simulink model "PubIfDecisionTOS_MDL"  (R2020b)
settings: configuration reference "DspaceConfig" (kept outside this file)
PostLoadFcn:
  | if any(exist('dsrtsu_mdlpostloadfcn', 'file') ~= 0), dsrtsu_mdlpostloadfcn('Execute', bdroot); end
InitFcn:
  | , if any(exist('dsmpb_private', 'file') ~= 0), dsmpb_private('dsmpb_mdlclblib', 'Init', bdroot); end,
undefined symbols (not defined in the file or in its folder): C_TOS_ACCEgoRAxletoFbumplength_m, C_TOS_ACCTargetFront_Flag, C_TOS_AEBJAPedObjDxThre_Val, C_TOS_AEBJAPedObjDyThre_Val, C_TOS_AEBJATargetSize_Val, C_TOS_AEBJAVehObjDxThre_Val, C_TOS_AEBJAVehObjDyThre_Val, C_TOS_AEBJuncPedTargetSize_Val, C_TOS_AEBLatObjDxThre_Val, C_TOS_AEBLatPedDyThre_Val, C_TOS_AEBLatTargetSize_Val, C_TOS_AEBLongTargetInEgoFront_Flag, C_TOS_axAbsGround_Parameter, C_TOS_CameraConfirmedFlag, C_TOS_CNsubjWidth, C_TOS_CurrentLaneCoreMinWidth_Val, C_TOS_CutInProb_Val_Zero, C_TOS_CutOutProb_Val_Zero, C_TOS_D2R_Val, C_TOS_DefaultValueObjectToCenterLine_dy, C_TOS_EgoCarWidth_Val, C_TOS_EgoDxRefPoint_m, C_TOS_EgoRAxletoFbumplength_m, C_TOS_HalfWidthVehicle_Con, C_TOS_HWA_CurrentLaneFlag, C_TOS_HWA_LeftLaneFlag, C_TOS_HWA_MovingDir_Vaild, C_TOS_HWA_MovState_Vaild, C_TOS_HWA_RightLaneFlag, C_TOS_LaneLineCourseErrorFront, C_TOS_LaneLineCourseErrorRear, C_TOS_MotorbikeDefaultWidth_m, C_TOS_NumberOfEffectiveTargets, C_TOS_Obj_Age_Val, C_TOS_Objdx_Constraint_Val, C_TOS_ObjectDefaultWidth_m, C_TOS_ObjInCurrentLane_Val, C_TOS_ObjInCurrentLaneValid, C_TOS_ObjInLeftLaneValid, C_TOS_ObjInRightLaneValid, C_TOS_ObjNotInCurrentLane_Val, C_TOS_ObjNotREElementType, C_TOS_ObjPredictDis_dy_ConstantVal_Zeros, C_TOS_ObjToCenterLine_ConstantVal_Zeros, C_TOS_OFMObjIDInvilad_Val, C_TOS_PIL_LatDisCons_Val_zero, C_TOS_PIL_ObjectCutInFlag_b, C_TOS_PIL_ObjectCutOutFlag_b, C_TOS_PIL_ObjLaneProb_al_Val, C_TOS_PP_ObjFusType_FC_Confirm_b, C_TOS_PP_ObjFusType_FC_FR_Confirm_b, C_TOS_PP_ObjFusType_FR_Confirm_b, C_TOS_RE_80BoolDefault_Val, C_TOS_RE_80Single181Default_Val, C_TOS_RE_80Single255Default_Val, C_TOS_RE_80Uint8Default_Val, C_TOS_RE_D2R, C_TOS_RE_D_180_Val, C_TOS_RE_InvalidObjectID_Val, C_TOS_RE_InvalidTargetChainDir_Val ... (+142)
libraries: simulink x1650, TOS_LIB x361, canfdmsglib x14
(part 8 of 69)

== system PubIfDecisionTOS_MDL/TOS_20201112/TOS_2012080320/TOS/AEB/TOS_AEBLatCro_20201208 ==
  TOSAAt_OFM_TIL_VIE : Inport
  AEBLatTrgInfor : Subsystem
  AEBLat_Object_Condition : Subsystem
  AEBLat_Object_Condition2 : Subsystem  Commented=on
  AEBLat_TargetIndex : Subsystem
  Bus Creator : BusCreator  Inputs=4
  Bus Selector1 : BusSelector  OutputSignals=OFM_SignalVerification.Object_ID,TOS_AddAttributes.PP_ObjFusType_FC_FR_Confirm,TOS_AddAttributes.PP_ObjFusType_FR_Confirm,OFM_SignalVerification.Object_Type,OFM_SignalVerification.Object_DX,OFM_SignalVerification.Object_DY,TOS_AddAttributes.PP_ObjMovingDirSignalProcessing,OFM_SignalVerification.Object_HeadingAngle,OFM_SignalVerification.Object_VX,OFM_SignalVerification.Object_VY,VIE_SignalVerification.vxvRefMs,VIE_SignalVerification.psiDtOpt
  Bus Selector2 : BusSelector  OutputSignals=OFM_SignalVerification,TOS_AddAttributes
  Bus Selector4 : BusSelector  Commented=on  OutputSignals=OFM_SignalVerification.Object_ID,TOS_AddAttributes.PP_ObjFusType_FC_FR_Confirm,TOS_AddAttributes.PP_ObjFusType_FR_Confirm,OFM_SignalVerification.Object_Type,OFM_SignalVerification.Object_DX,OFM_SignalVerification.Object_DY,TOS_AddAttributes.PP_ObjMovingDirSignalProcessing,OFM_SignalVerification.Object_HeadingAngle,OFM_SignalVerification.Object_VX,OFM_SignalVerification.Object_VY,VIE_SignalVerification.vxvRefMs,VIE_SignalVerification.psiDtOpt
  Display{5..9} (5 alike) : Display  Commented=on
  From2 : From  Commented=on  GotoTag=TOS_AEB_LATOBJ
  Selector{10..19} (10 alike) : Selector  Commented=on  InputPortWidth=80  IndexOptions=Index vector (dialog)  Indices=64  OutputSizes=1
  Subsystem : Subsystem
  Subsystem1 : Subsystem
  Subsystem2 : Subsystem  Commented=on
  Terminator : Terminator
  Unit Delay{,1,3..4} (4 alike) : UnitDelay  SampleTime=-1  HasFrameUpgradeWarning=on
  Unit Delay2 : UnitDelay  Commented=on  SampleTime=-1  HasFrameUpgradeWarning=on
  TOS_AEB_LATOBJ : Outport
  wires:
  Bus Selector1/3 -> AEBLat_Object_Condition/3(PP_ObjFusType_FR_Confirm)  "<PP_ObjFusType_FR_Confirm>"
  Bus Selector1/2 -> AEBLat_Object_Condition/2(PP_ObjFusType_FC_FR_Confirm)  "<PP_ObjFusType_FC_FR_Confirm>"
  Bus Selector1/11 -> AEBLat_Object_Condition/11(VIE_EgoVelocity)  "<vxvRefMs>"
  Bus Selector1/10 -> AEBLat_Object_Condition/10(Object_VY)  "<Object_VY>"
  Bus Selector1/9 -> AEBLat_Object_Condition/9(Object_VX)  "<Object_VX>"
  Bus Selector1/8 -> AEBLat_Object_Condition/8(Object_HeadingAngle)  "<Object_HeadingAngle>"
  Bus Selector1/7 -> AEBLat_Object_Condition/7(PP_ObjMovingDirSignalProcessing)  "<PP_ObjMovingDirSignalProcessing>"
  Bus Selector1/1 -> AEBLat_Object_Condition/1(Object_ID)  "<Object_ID>"
  Bus Selector1/4 -> AEBLat_Object_Condition/4(ObjectType)  "<Object_Type>"
  Bus Selector2/1 -> AEBLatTrgInfor/1(OFM_SignalVerification)  "<OFM_SignalVerification>"
  Bus Selector2/2 -> AEBLatTrgInfor/2(TOS_AddAttributes)  "<TOS_AddAttributes>"
  Bus Selector1/5 -> AEBLat_Object_Condition/5(Object_Dx)  "<Object_DX>"
  Bus Selector1/6 -> AEBLat_Object_Condition/6(Object_Dy)  "<Object_DY>"
  AEBLat_TargetIndex/1(AEBLat_Target_Index) -> AEBLatTrgInfor/3(TOS_AEBLatTrg_Index)  "TOS_AEBLat_Index"
  AEBLat_Object_Condition/1(TOS_AEBLat_ConditionTargets_Dx) -> AEBLat_TargetIndex/1(TOS_AEBLat_Targets_Dx)  "TOS_AEBLat_ConditionTargets_Dx"
  AEBLat_Object_Condition/2(AEBLat_TargetFusionType_observal) -> Bus Creator/1  "TOS_AEBLat_TargetFusionType_observal"
  AEBLat_Object_Condition/3(AEBLat_TargetObjectType_observal) -> Bus Creator/2  "TOS_AEBLat_TargetObjectType_observal"
  AEBLat_Object_Condition/4(AEBLat_TargetDXDY_observal) -> Bus Creator/3  "TOS_AEBLat_TargetDXDY_observal"
  AEBLat_Object_Condition/5(AEBLat_TargetMovDir_observal) -> Bus Creator/4  "TOS_AEBLat_TargetMovDir_observal"
  AEBLatTrgInfor/1(TOS_AEB_LATOBJ) -> [TOS_AEB_LATOBJ], TOS_AEB_LATOBJ/1
  Bus Selector1/12 -> AEBLat_Object_Condition/12(psiDtOpt)  "<psiDtOpt>"
  [TOS_AEB_LATOBJ] -> Subsystem/1(TOS_AEB_LATOBJ)
  Subsystem/1(ObjectID) -> Unit Delay/1
  Unit Delay/1 -> AEBLat_Object_Condition/13(AEBLat_Target_ObjectID_K1)
  Selector18/1 -> AEBLat_Object_Condition2/9(Object_VX)
  Selector19/1 -> AEBLat_Object_Condition2/10(Object_VY)
  Selector16/1 -> AEBLat_Object_Condition2/7(PP_ObjMovingDirSignalProcessing)
  Selector17/1 -> AEBLat_Object_Condition2/8(Object_HeadingAngle)
  Selector15/1 -> AEBLat_Object_Condition2/6(Object_Dy)
  Selector14/1 -> AEBLat_Object_Condition2/5(Object_Dx)
  Selector13/1 -> AEBLat_Object_Condition2/4(ObjectType)
  Selector12/1 -> AEBLat_Object_Condition2/3(PP_ObjFusType_FR_Confirm)
  Selector11/1 -> AEBLat_Object_Condition2/2(PP_ObjFusType_FC_FR_Confirm)
  Selector10/1 -> AEBLat_Object_Condition2/1(Object_ID)
  Bus Selector4/3 -> Selector12/1  "<PP_ObjFusType_FR_Confirm>"
  Bus Selector4/2 -> Selector11/1  "<PP_ObjFusType_FC_FR_Confirm>"
  Bus Selector4/11 -> AEBLat_Object_Condition2/11(VIE_EgoVelocity)  "<vxvRefMs>"
  Bus Selector4/10 -> Selector19/1  "<Object_VY>"
  Bus Selector4/9 -> Selector18/1  "<Object_VX>"
  Bus Selector4/8 -> Selector17/1  "<Object_HeadingAngle>"
  Bus Selector4/7 -> Selector16/1  "<PP_ObjMovingDirSignalProcessing>"
  Bus Selector4/1 -> Selector10/1  "<Object_ID>"
  Bus Selector4/4 -> Selector13/1  "<Object_Type>"
  Bus Selector4/5 -> Selector14/1  "<Object_DX>"
  Bus Selector4/6 -> Selector15/1  "<Object_DY>"
  TOSAAt_OFM_TIL_VIE/1 -> Bus Selector2/1, Bus Selector4/1, Bus Selector1/1
  Bus Selector4/12 -> AEBLat_Object_Condition2/12(psiDtOpt)  "<psiDtOpt>"
  From2/1 -> Subsystem2/1(TOS_AEB_LATOBJ)
  Subsystem2/1(ObjectID) -> Unit Delay2/1
  Unit Delay2/1 -> AEBLat_Object_Condition2/13(AEBLat_Target_ObjectID_K1)
  AEBLat_Object_Condition2/5(AEBLat_TargetMovDir_observal) -> Display9/1
  AEBLat_Object_Condition2/4(AEBLat_TargetDXDY_observal) -> Display8/1
  AEBLat_Object_Condition2/3(AEBLat_TargetObjectType_observal) -> Display7/1
  AEBLat_Object_Condition2/2(AEBLat_TargetFusionType_observal) -> Display6/1
  AEBLat_Object_Condition2/1(TOS_AEBLat_ConditionTargets_Dx) -> Display5/1
  Subsystem/2(ObjectType) -> Unit Delay3/1
  Unit Delay3/1 -> AEBLat_Object_Condition/14(AEBLat_Target_ObjectType_K1)
  Unit Delay4/1 -> AEBLatTrgInfor/5(AEBLat_Target_ObjectType_K1)
  Subsystem1/2(ObjectType) -> Unit Delay4/1
  Unit Delay1/1 -> AEBLatTrgInfor/4(AEBLat_Target_ObjectID_K1)
  Subsystem1/1(ObjectID) -> Unit Delay1/1
  [TOS_AEB_LATOBJ] -> Subsystem1/1(TOS_AEB_LATOBJ)
  Bus Creator/1 -> Terminator/1  "TOS_AEBLat_ObserVal"

== system PubIfDecisionTOS_MDL/TOS_20201112/TOS_2012080320/TOS/AEB/TOS_AEBLong ==
  note: 目标分裂，去除Dx2米之内的分裂目标
  TOSAAt_OFM_TIL_VIE : Inport
  AEBLongTargetInfor : Subsystem
  AEBLong_Confirm : Subsystem
  AEBLong_Target_PreJudge : Subsystem
  Bus Selector : BusSelector  OutputSignals=ObjectID,dx
  Bus Selector2 : BusSelector  OutputSignals=OFM_SignalVerification,TOS_AddAttributes
  Bus Selector3 : BusSelector  OutputSignals=OFM_SignalVerification.Object_DX,OFM_SignalVerification.Object_ID,TLJ_TargetInLaneValidityJudg.TOS_TLJ_SameLaneConfirm_Flag
  Bus Selector4 : BusSelector  OutputSignals=VIE_SignalVerification.vxvRefMs,OFM_SignalVerification,TOS_AddAttributes,TLJ_TargetInLaneValidityJudg,PP_CenterLineCalculat,TOS_ProbInLaneCalculat,TOS_VCAN_SignalVerification,TOS_ProbInLaneCalculat.PIL_OverlapRatio
  Bus Selector5 : BusSelector  OutputSignals=TOS_AddAttributes.PP_ObjFusType_FC_FR_Confirm,TOS_AddAttributes.PP_ObjFusType_FR_Confirm,TOS_AddAttributes.PP_ObjFusType_FC_Confirm,OFM_SignalVerification.Object_ID,OFM_SignalVerification.Object_MovingState,OFM_SignalVerification.Object_DX,OFM_SignalVerification.Object_ObstacleProb,OFM_SignalVerification.Object_DY,PP_REElementType
  Bus Selector6 : BusSelector  OutputSignals=ObjectID,ObjectMovingState
  Constant2 : Constant  Value=C_TOS_NumberOfEffectiveTargets  OutDataTypeStr=uint8
      settings: AttributesFormatString=C_TOS_NumberOfEffectiveTargets = 80
  Delay : Delay  InitialCondition=0
  Delay1 : Delay  DelayLength=1  InitialCondition=0
  Delay2 : Delay  InitialCondition=0
  Delay3 : Delay  DelayLength=1  InitialCondition=0
  MATLAB Function1 : MATLAB Function  TreatAsAtomicUnit=on
  MATLAB Function2 : MATLAB Function  Commented=on  TreatAsAtomicUnit=on
  Terminator : Terminator
  Terminator1 : Terminator
  Terminator2 : Terminator
  Unit Delay : UnitDelay  SampleTime=-1  HasFrameUpgradeWarning=on
  Unit Delay1 : UnitDelay  InitialCondition=255  SampleTime=-1  HasFrameUpgradeWarning=on
  TOS_AEBLONOBJ : Outport
  wires:
  Bus Selector4/4 -> AEBLong_Confirm/4(TLJ_TargetInLaneValidityJudg)  "<TLJ_TargetInLaneValidityJudg>"
  Bus Selector4/3 -> AEBLong_Confirm/3(TOS_AddAttributes)  "<TOS_AddAttributes>"
  Bus Selector4/2 -> AEBLong_Confirm/2(OFM_SignalVerification)  "<OFM_SignalVerification>"
  Bus Selector4/1 -> AEBLong_Confirm/1(VIE_EgoVelocity)  "<vxvRefMs>"
  Bus Selector2/2 -> AEBLongTargetInfor/2(TOS_AddAttributes)  "<TOS_AddAttributes>"
  AEBLongTargetInfor/1(TOS_AEBLONOBJ) -> [TOS_AEBLONOBJ], TOS_AEBLONOBJ/1
  Bus Selector2/1 -> AEBLongTargetInfor/1(OFM_SignalVerification)  "<OFM_SignalVerification>"
  AEBLong_Confirm/1(TOS_AEBLong_TargetIndex) -> AEBLongTargetInfor/3(TOS_AEBLongTargetIndex)
  Bus Selector4/5 -> AEBLong_Confirm/5(PP_CenterLineCalculat)  "<PP_CenterLineCalculat>"
  Bus Selector4/6 -> AEBLong_Confirm/6(PIL_ProbInLaneCalculat)  "<TOS_ProbInLaneCalculat>"
  Bus Selector4/7 -> AEBLong_Confirm/7(<TOS_VCAN_SignalVerification>)  "<TOS_VCAN_SignalVerification>"
  Bus Selector3/1 -> MATLAB Function1/1(Object_Dx)  "<Object_DX>"
  Bus Selector3/2 -> MATLAB Function1/2(Object_ID)  "<Object_ID>"
  MATLAB Function1/1(Dx1stNearestObjIndex) -> AEBLong_Confirm/9(AEBLong_Index)  "TOS_AEBLong_Index"
  MATLAB Function1/2(Dx1stNearestObjID) -> Terminator/1
  MATLAB Function1/3(Dx2edNearestObjIndex) -> Terminator1/1
  MATLAB Function1/4(Dx2edNearestObjID) -> Terminator2/1
  Constant2/1 -> MATLAB Function1/5(Object_Num)
  Bus Selector3/3 -> MATLAB Function1/3(ConditionJudge)  "<TOS_TLJ_SameLaneConfirm_Flag>"
  Bus Selector4/8 -> AEBLong_Confirm/8(PIL_OverlapRatio)  "<PIL_OverlapRatio>"
  Unit Delay1/1 -> AEBLong_Target_PreJudge/11(AEBLONG_TargetP0_Dx_K1)
  TOSAAt_OFM_TIL_VIE/1 -> Bus Selector5/1, Bus Selector2/1, Bus Selector4/1, Bus Selector3/1
  [TOS_AEBLONOBJ] -> Bus Selector/1
  Bus Selector/2 -> Unit Delay1/1  "<dx>"
  Bus Selector/1 -> Unit Delay/1  "<ObjectID>"
  Unit Delay/1 -> AEBLong_Target_PreJudge/10(AEBLONG_TargetP0_ID_K1)
  AEBLong_Target_PreJudge/1(TOS_AEBLONG_TargetPreFiltFlag) -> MATLAB Function1/4(TargetFusionTypeFlag)  "TOS_AEBLONG_TargetPreFiltFlag"
  Bus Selector6/2 -> Delay3/1, Delay2/1  "<ObjectMovingState>"
  [TOS_AEBLONOBJ] -> Bus Selector6/1
  Bus Selector6/1 -> Delay1/1, Delay/1  "<ObjectID>"
  Delay1/1 -> AEBLong_Confirm/10(AEBLong_Target_ID_K1)
  Delay/1 -> AEBLong_Confirm/11(AEBLong_Target_ID_K2)
  Delay3/1 -> AEBLong_Confirm/12(AEBLong_Target_MovState_K1)
  Delay2/1 -> AEBLong_Confirm/13(AEBLong_Target_MovState_K2)
  Bus Selector5/1 -> AEBLong_Target_PreJudge/1(PP_ObjFusType_FC_FR_Confirm)  "<PP_ObjFusType_FC_FR_Confirm>"
  Bus Selector5/2 -> AEBLong_Target_PreJudge/2(PP_ObjFusType_FR_Confirm)  "<PP_ObjFusType_FR_Confirm>"
  Bus Selector5/3 -> AEBLong_Target_PreJudge/3(PP_ObjFusType_FC_Confirm)  "<PP_ObjFusType_FC_Confirm>"
  Bus Selector5/4 -> AEBLong_Target_PreJudge/4(Object_ID)  "<Object_ID>"
  Bus Selector5/5 -> AEBLong_Target_PreJudge/5(Obj_MovingState)  "<Object_MovingState>"
  Bus Selector5/6 -> AEBLong_Target_PreJudge/6(Obj_Dx)  "<Object_DX>"
  Bus Selector5/7 -> AEBLong_Target_PreJudge/7(Object_ObstacleProb)  "<Object_ObstacleProb>"
  Bus Selector5/8 -> AEBLong_Target_PreJudge/8(Object_DY)  "<Object_DY>"
  Bus Selector5/9 -> AEBLong_Target_PreJudge/9(PP_REElementType)  "<PP_REElementType>"

== system PubIfDecisionTOS_MDL/TOS_20201112/TOS_2012080320/TOS/LC_LCKie_ELK/ELK_TargetInfor ==
  TOS_HWA_TargetIndexVector : Inport
  TOSAAt_OFM_TIL_VIE : Inport  Port=2
  ObjectIn_Lane_b : Inport  Port=3
  Bus Creator : BusCreator  Inputs=3
  Bus Selector2 : BusSelector  OutputSignals=TOSAAt_OFM_TIL_VIE.OFM_SignalVerification,TOSAAt_OFM_TIL_VIE.TOS_AddAttributes,TOSAAt_OFM_TIL_VIE.TOS_ProbInLaneCalculat,ObjectIn_Lane_b
  Bus Selector5 : BusSelector  OutputSignals=TOS_HWA_TargetIndexVector
  TOS_ELKTargetInfor : Stateflow chart  TreatAsAtomicUnit=on
  TOS_ELKTarget : Outport
  wires:
  Bus Selector2/4 -> TOS_ELKTargetInfor/4(ObjectIn_Lane_b)  "<ObjectIn_Lane_b>"
  ObjectIn_Lane_b/1 -> Bus Creator/3  "ObjectIn_Lane_b"
  Bus Selector5/1 -> TOS_ELKTargetInfor/5(TOS_HWA_TargetIndexVector)  "<TOS_HWA_TargetIndexVector>"
  TOSAAt_OFM_TIL_VIE/1 -> Bus Creator/1  "TOSAAt_OFM_TIL_VIE"
  TOS_HWA_TargetIndexVector/1 -> Bus Creator/2  "TOS_HWA_TargetIndexVector"
  Bus Selector2/3 -> TOS_ELKTargetInfor/3(TOS_ProbInLaneCalculat)  "<TOS_ProbInLaneCalculat>"
  Bus Selector2/2 -> TOS_ELKTargetInfor/2(TOS_AddAttributes)  "<TOS_AddAttributes>"
  Bus Selector2/1 -> TOS_ELKTargetInfor/1(OFM_SignalVerification)  "<OFM_SignalVerification>"
  TOS_ELKTargetInfor/1(TOS_ELKTargetInfor) -> TOS_ELKTarget/1
  Bus Creator/1 -> Bus Selector5/1, Bus Selector2/1

== system PubIfDecisionTOS_MDL/TOS_20201112/TOS_2012080320/TOS/LC_LCKie_ELK/HWA_TargetInfor ==
  TOS_HWA_TargetIndexVector : Inport
  TOSAAt_OFM_TIL_VIE : Inport  Port=2
  ObjectIn_Lane_b : Inport  Port=3
  Bus Creator : BusCreator  Inputs=3
  Bus Selector : BusSelector  OutputSignals=TOSAAt_OFM_TIL_VIE.OFM_SignalVerification,TOSAAt_OFM_TIL_VIE.TOS_AddAttributes,TOSAAt_OFM_TIL_VIE.TOS_ProbInLaneCalculat,ObjectIn_Lane_b
  Bus Selector4 : BusSelector  OutputSignals=TOS_HWA_TargetIndexVector
  TOS_HWA_TargetInfor : Stateflow chart  TreatAsAtomicUnit=on
  TOS_HWA_Target : Outport
  wires:
  Bus Selector/4 -> TOS_HWA_TargetInfor/4(ObjectIn_Lane_b)  "<ObjectIn_Lane_b>"
  ObjectIn_Lane_b/1 -> Bus Creator/3  "ObjectIn_Lane_b"
  Bus Selector4/1 -> TOS_HWA_TargetInfor/5(TOS_HWA_TargetIndexVector)  "<TOS_HWA_TargetIndexVector>"
  TOSAAt_OFM_TIL_VIE/1 -> Bus Creator/1  "TOSAAt_OFM_TIL_VIE"
  TOS_HWA_TargetIndexVector/1 -> Bus Creator/2  "TOS_HWA_TargetIndexVector"
  Bus Creator/1 -> Bus Selector/1, Bus Selector4/1
  Bus Selector/3 -> TOS_HWA_TargetInfor/3(TOS_ProbInLaneCalculat)  "<TOS_ProbInLaneCalculat>"
  Bus Selector/2 -> TOS_HWA_TargetInfor/2(TOS_AddAttributes)  "<TOS_AddAttributes>"
  Bus Selector/1 -> TOS_HWA_TargetInfor/1(OFM_SignalVerification)  "<OFM_SignalVerification>"
  TOS_HWA_TargetInfor/1(TOS_LCTargetInfor) -> TOS_HWA_Target/1

== system PubIfDecisionTOS_MDL/TOS_20201112/TOS_2012080320/TOS/LC_LCKie_ELK/LCKie_TargetInfor ==
  TOS_HWA_TargetIndexVector : Inport
  TOSAAt_OFM_TIL_VIE : Inport  Port=2
  ObjectIn_Lane_b : Inport  Port=3
  Bus Creator : BusCreator  Inputs=3
  Bus Selector1 : BusSelector  OutputSignals=TOSAAt_OFM_TIL_VIE.OFM_SignalVerification,TOSAAt_OFM_TIL_VIE.TOS_AddAttributes,TOSAAt_OFM_TIL_VIE.TOS_ProbInLaneCalculat,ObjectIn_Lane_b
  Bus Selector3 : BusSelector  OutputSignals=TOS_HWA_TargetIndexVector
  TOS_LCKieTargetInfor : Stateflow chart  TreatAsAtomicUnit=on
  TOS_LCKIETarget : Outport
  wires:
  Bus Creator/1 -> Bus Selector3/1, Bus Selector1/1
  TOS_LCKieTargetInfor/1(TOS_LCKieTargetInfor) -> TOS_LCKIETarget/1
  Bus Selector1/1 -> TOS_LCKieTargetInfor/1(OFM_SignalVerification)  "<OFM_SignalVerification>"
  Bus Selector1/2 -> TOS_LCKieTargetInfor/2(TOS_AddAttributes)  "<TOS_AddAttributes>"
  Bus Selector1/3 -> TOS_LCKieTargetInfor/3(TOS_ProbInLaneCalculat)  "<TOS_ProbInLaneCalculat>"
  TOS_HWA_TargetIndexVector/1 -> Bus Creator/2  "TOS_HWA_TargetIndexVector"
  TOSAAt_OFM_TIL_VIE/1 -> Bus Creator/1  "TOSAAt_OFM_TIL_VIE"
  Bus Selector3/1 -> TOS_LCKieTargetInfor/5(TOS_HWA_TargetIndexVector)  "<TOS_HWA_TargetIndexVector>"
  ObjectIn_Lane_b/1 -> Bus Creator/3  "ObjectIn_Lane_b"
  Bus Selector1/4 -> TOS_LCKieTargetInfor/4(ObjectIn_Lane_b)  "<ObjectIn_Lane_b>"

== system PubIfDecisionTOS_MDL/TOS_20201112/TOS_2012080320/TOS/LC_LCKie_ELK/TOS_HWA ==
  TOSAAt_OFM_TIL_VIE : Inport
  TOS_HWA_CurrentFront_Target_2 : Inport  Port=2
  CurrentLane : Subsystem
  LeftLane : Subsystem
  RightLane : Subsystem
  Vector Concatenate3 : Concatenate  NumInputs=3
  HWA_LeftFront_Target_1 : Outport
  HWA_LeftFront_Target_2 : Outport  Port=2
  HWA_LeftRear_Target_3 : Outport  Port=3
  HWA_LeftRear_Target_4 : Outport  Port=4
  HWA_RightFront_Target_1 : Outport  Port=5
  HWA_RightFront_Target_2 : Outport  Port=6
  HWA_RightRear_Target_3 : Outport  Port=7
  HWA_RightRear_Target_4 : Outport  Port=8
  HWA_CurrentFront_Target_1 : Outport  Port=9
  HWA_CurrentFront_Target_2 : Outport  Port=10
  HWA_CurrentRear_Target_3 : Outport  Port=11
  ObjectIn_Lane_b : Outport  Port=12
  wires:
  TOS_HWA_CurrentFront_Target_2/1 -> CurrentLane/2(TOS_HWA_CurrentFront_Target_2)
  CurrentLane/1(HWA_CurrentFront_Target_1) -> HWA_CurrentFront_Target_1/1
  CurrentLane/2(HWA_CurrentFront_Target_2) -> HWA_CurrentFront_Target_2/1
  CurrentLane/3(HWA_CurrentRear_Target_3) -> HWA_CurrentRear_Target_3/1
  Vector Concatenate3/1 -> ObjectIn_Lane_b/1
  RightLane/1(HWA_RightFront_Target_1) -> HWA_RightFront_Target_1/1
  RightLane/2(HWA_RightFront_Target_2) -> HWA_RightFront_Target_2/1
  RightLane/3(HWA_RightRear_Target_3) -> HWA_RightRear_Target_3/1
  RightLane/4(HWA_RightRear_Target_4) -> HWA_RightRear_Target_4/1
  LeftLane/1(HWA_LeftFront_Target_1) -> HWA_LeftFront_Target_1/1
  LeftLane/2(HWA_LeftFront_Target_2) -> HWA_LeftFront_Target_2/1
  LeftLane/3(HWA_LeftRear_Target_3) -> HWA_LeftRear_Target_3/1
  LeftLane/4(HWA_LeftRear_Target_4) -> HWA_LeftRear_Target_4/1
  TOSAAt_OFM_TIL_VIE/1 -> CurrentLane/1(TOSAAt_OFM_TIL_VIE), RightLane/1(TOSAAt_OFM_TIL_VIE), LeftLane/1(TOSAAt_OFM_TIL_VIE)
  LeftLane/5(TargetInLeftLane_b) -> [TargetInLeftLane_b]
  RightLane/5(TargetInRightLane_b) -> [TargetInRightLane_b]
  [TargetInLeftLane_b] -> Vector Concatenate3/1
  [TargetInRightLane_b] -> Vector Concatenate3/2
  CurrentLane/4(TargetInCurrentLane_b) -> [TargetInCurrentLane_b]
  [TargetInCurrentLane_b] -> Vector Concatenate3/3

== system PubIfDecisionTOS_MDL/TOS_20201112/TOS_2012080320/TOS/OutPutPortAdaptation/OFM_PortAdaptation ==
  OFMInfo : Inport
  Bus Creator1 : BusCreator  Inputs=29
  Bus Selector : BusSelector  OutputSignals=Object_Fus_Type,Object_ID,Object_Type,Object_Length,Object_Width,Object_Hight,Object_HeadingAngle,Object_YawAngle,Object_MovingState,Object_Orientation,Object_DX,Object_DY,Object_VX,Object_VY,Object_Std_AX,Object_Std_AY,Object_Std_DX,Object_Std_DY,Object_Std_VX,Object_Std_VY,Object_AX,Object_AY,Object_Std_Length,Object_Std_Width,Object_Std_HeadingAngle,Object_Type_Prob,Object_ExistProb,Object_ObstacleProb,Object_Age
  Signal Copy{,1..20,24..31} (29 alike) : SignalConversion  OverrideOpt=off
  OFM_SignalVerification : Outport
  wires:
  Bus Creator1/1 -> OFM_SignalVerification/1  "OFM_SignalVerification"
  Signal Copy25/1 -> Bus Creator1/20  "Object_Std_VY"
  Signal Copy10/1 -> Bus Creator1/11  "Object_DX"
  Signal Copy27/1 -> Bus Creator1/22  "Object_AY"
  Signal Copy16/1 -> Bus Creator1/17  "Object_Std_DX"
  Signal Copy13/1 -> Bus Creator1/14  "Object_VY"
  Signal Copy26/1 -> Bus Creator1/21  "Object_AX"
  Signal Copy15/1 -> Bus Creator1/16  "Object_Std_AY"
  Signal Copy7/1 -> Bus Creator1/8  "Object_YawAngle"
  Signal Copy24/1 -> Bus Creator1/19  "Object_Std_VX"
  Signal Copy4/1 -> Bus Creator1/5  "Object_Width"
  Signal Copy29/1 -> Bus Creator1/24  "Object_Std_Width"
  Signal Copy20/1 -> Bus Creator1/29  "Object_Age"
  Signal Copy18/1 -> Bus Creator1/27  "Object_ExistProb"
  Signal Copy28/1 -> Bus Creator1/23  "Object_Std_Length"
  Signal Copy6/1 -> Bus Creator1/7  "Object_HeadingAngle"
  Signal Copy12/1 -> Bus Creator1/13  "Object_VX"
  Signal Copy11/1 -> Bus Creator1/12  "Object_DY"
  Signal Copy30/1 -> Bus Creator1/25  "Object_Std_HeadingAngle"
  Signal Copy2/1 -> Bus Creator1/3  "Object_Type"
  Signal Copy5/1 -> Bus Creator1/6  "Object_Hight"
  Signal Copy/1 -> Bus Creator1/1  "Object_Fus_Type"
  Signal Copy14/1 -> Bus Creator1/15  "Object_Std_AX"
  Signal Copy9/1 -> Bus Creator1/10  "Object_Orientation"
  Signal Copy19/1 -> Bus Creator1/28  "Object_ObstacleProb"
  Signal Copy31/1 -> Bus Creator1/26  "Object_Type_Prob"
  Signal Copy8/1 -> Bus Creator1/9  "Object_MovingState"
  Signal Copy3/1 -> Bus Creator1/4  "Object_Length"
  Signal Copy1/1 -> Bus Creator1/2  "Object_ID"
  Signal Copy17/1 -> Bus Creator1/18  "Object_Std_DY"
  Bus Selector/29 -> Signal Copy20/1  "<Object_Age>"
  Bus Selector/28 -> Signal Copy19/1  "<Object_ObstacleProb>"
  Bus Selector/27 -> Signal Copy18/1  "<Object_ExistProb>"
  Bus Selector/26 -> Signal Copy31/1  "<Object_Type_Prob>"
  Bus Selector/25 -> Signal Copy30/1  "<Object_Std_HeadingAngle>"
  Bus Selector/24 -> Signal Copy29/1  "<Object_Std_Width>"
  Bus Selector/23 -> Signal Copy28/1  "<Object_Std_Length>"
  Bus Selector/22 -> Signal Copy27/1  "<Object_AY>"
  Bus Selector/21 -> Signal Copy26/1  "<Object_AX>"
  Bus Selector/20 -> Signal Copy25/1  "<Object_Std_VY>"
  Bus Selector/19 -> Signal Copy24/1  "<Object_Std_VX>"
  Bus Selector/18 -> Signal Copy17/1  "<Object_Std_DY>"
  Bus Selector/17 -> Signal Copy16/1  "<Object_Std_DX>"
  Bus Selector/13 -> Signal Copy12/1  "<Object_VX>"
  Bus Selector/14 -> Signal Copy13/1  "<Object_VY>"
  Bus Selector/15 -> Signal Copy14/1  "<Object_Std_AX>"
  Bus Selector/16 -> Signal Copy15/1  "<Object_Std_AY>"
  Bus Selector/12 -> Signal Copy11/1  "<Object_DY>"
  Bus Selector/11 -> Signal Copy10/1  "<Object_DX>"
  Bus Selector/10 -> Signal Copy9/1  "<Object_Orientation>"
  Bus Selector/9 -> Signal Copy8/1  "<Object_MovingState>"
  Bus Selector/8 -> Signal Copy7/1  "<Object_YawAngle>"
  Bus Selector/7 -> Signal Copy6/1  "<Object_HeadingAngle>"
  Bus Selector/6 -> Signal Copy5/1  "<Object_Hight>"
  Bus Selector/5 -> Signal Copy4/1  "<Object_Width>"
  Bus Selector/4 -> Signal Copy3/1  "<Object_Length>"
  Bus Selector/3 -> Signal Copy2/1  "<Object_Type>"
  Bus Selector/2 -> Signal Copy1/1  "<Object_ID>"
  Bus Selector/1 -> Signal Copy/1  "<Object_Fus_Type>"
  OFMInfo/1 -> Bus Selector/1  "OFMInfo"

== system PubIfDecisionTOS_MDL/TOS_20201112/TOS_2012080320/TOS/P0_Trajectory_V1.0/CordinatConvert ==
  note: P0参数，初始默认设置
  VehStandstill : Inport
  PsiDtOpt : Inport  Port=2
  VxvRef_ms : Inport  Port=3
  P0_TrackRecord_K1 : Inport  Port=4
  Bus Creator : BusCreator  Inputs=4
  Bus Creator1 : BusCreator  Inputs=3
  Bus Selector : BusSelector  OutputSignals=PsiDtOpt,VxvRef_ms
  Bus Selector1 : BusSelector  OutputSignals=EgoVeh_OffsetX,EgoVeh_OffsetY,EgoVeh_OffsetAngle
  Bus Selector2 : BusSelector  OutputSignals=VxvRef_ms,VehStandstill,P0_TrackRecord_K1.P0_dx_TrackRecord,P0_TrackRecord_K1.P0_dy_TrackRecord,P0_TrackRecord_K1.P0_Counter_TrackRecord,P0_TrackRecord_K1.P0_ID_TrackRecord
  CordinatConvert : Subsystem
  CordinatConvert1 : Subsystem  Commented=on
  EgoVehicleOffset : Subsystem
  Gain : Gain  Gain=-1
  Unit Delay1 : UnitDelay  InitialCondition=single(zeros(P_TOS_P0_Trajectory_TrackRecord_Num,1))  SampleTime=-1  HasFrameUpgradeWarning=on
  Unit Delay2 : UnitDelay  InitialCondition=single(zeros(P_TOS_P0_Trajectory_TrackRecord_Num,1))  SampleTime=-1  HasFrameUpgradeWarning=on
  Unit Delay3 : UnitDelay  InitialCondition=uint32(zeros(P_TOS_P0_Trajectory_TrackRecord_Num,1))  SampleTime=-1  HasFrameUpgradeWarning=on
  Unit Delay4 : UnitDelay  InitialCondition=uint8(zeros(P_TOS_P0_Trajectory_TrackRecord_Num,1))  SampleTime=-1  HasFrameUpgradeWarning=on
  P0_dx_TrackRecord_CordinatConvert_K1 : Outport
  P0_dy_TrackRecord_CordinatConvert_K1 : Outport  Port=2
  P0_Counter_TrackRecord_CordinatConvert_K1 : Outport  Port=3
  P0_ID_TrackRecord_CordinatConvert_K1 : Outport  Port=4
  wires:
  Unit Delay3/1 -> CordinatConvert/8(P0_Counter_TrackRecord_K1)
  Unit Delay1/1 -> CordinatConvert/7(P0_dy_TrackRecord_K1)
  Unit Delay2/1 -> CordinatConvert/6(P0_dx_TrackRecord_K1)
  CordinatConvert/3(P0_Counter_TrackRecord_CordinatConvert_K1) -> P0_Counter_TrackRecord_CordinatConvert_K1/1  "P0_Counter_TrackRecord_CordinatConvert_K1"
  CordinatConvert/2(P0_dy_TrackRecord_CordinatConvert_K1) -> P0_dy_TrackRecord_CordinatConvert_K1/1  "P0_dy_TrackRecord_CordinatConvert_K1"
  CordinatConvert/1(P0_dx_TrackRecord_CordinatConvert_K1) -> P0_dx_TrackRecord_CordinatConvert_K1/1  "P0_dx_TrackRecord_CordinatConvert_K1"
  Bus Selector2/5 -> Unit Delay3/1  "<P0_Counter_TrackRecord>"
  Bus Selector2/4 -> Unit Delay1/1  "<P0_dy_TrackRecord>"
  Bus Selector2/3 -> Unit Delay2/1  "<P0_dx_TrackRecord>"
  Bus Selector2/2 -> CordinatConvert/5(VehStandstill)  "<VehStandstill>"
  Bus Selector1/3 -> CordinatConvert/3(EgoVeh_OffsetAngle)  "<EgoVeh_OffsetAngle>"
  Bus Selector1/2 -> CordinatConvert/2(EgoVeh_OffsetY)  "<EgoVeh_OffsetY>"
  Bus Selector1/1 -> CordinatConvert/1(EgoVeh_OffsetX)  "<EgoVeh_OffsetX>"
  Bus Creator1/1 -> Bus Selector1/1
  EgoVehicleOffset/1(EgoVeh_OffsetX) -> Bus Creator1/1  "EgoVeh_OffsetX"
  Gain/1 -> Bus Creator1/3  "EgoVeh_OffsetAngle"
  EgoVehicleOffset/2(EgoVeh_OffsetY) -> Bus Creator1/2  "EgoVeh_OffsetY"
  Bus Selector/2 -> EgoVehicleOffset/2(VxvRef_ms)  "<VxvRef_ms>"
  Bus Selector/1 -> EgoVehicleOffset/1(PsiDtOpt)  "<PsiDtOpt>"
  Bus Creator/1 -> Bus Selector/1, Bus Selector2/1
  VxvRef_ms/1 -> Bus Creator/4  "VxvRef_ms"
  PsiDtOpt/1 -> Bus Creator/3  "PsiDtOpt"
  VehStandstill/1 -> Bus Creator/2  "VehStandstill"
  P0_TrackRecord_K1/1 -> Bus Creator/1  "P0_TrackRecord_K1"
  EgoVehicleOffset/3(EgoVeh_OffsetAngle) -> Gain/1
  CordinatConvert/4(P0_ID_TrackRecord_CordinatConvert_K1) -> P0_ID_TrackRecord_CordinatConvert_K1/1  "P0_ID_TrackRecord_CordinatConvert_K1"
  Bus Selector2/6 -> Unit Delay4/1  "<P0_ID_TrackRecord>"
  Unit Delay4/1 -> CordinatConvert/9(P0_ID_TrackRecord_K1)
  Bus Selector2/1 -> CordinatConvert/4(VxvRef_ms)  "<VxvRef_ms>"

== system PubIfDecisionTOS_MDL/TOS_20201112/TOS_2012080320/TOS/P0_Trajectory_V1.0/DataConfirm ==
  P0_TrackRecord : Inport
  Bus Selector : BusSelector  OutputSignals=P0_StartPosition_Num,P0_EndPosition_Num
  Bus Selector1 : BusSelector  OutputSignals=P0_StartPosition_Num,P0_EndPosition_Num
  Bus Selector2 : BusSelector  OutputSignals=P0_dx_TrackRecord,P0_dy_TrackRecord,P0_Counter_TrackRecord,P0_StartPosition_Num,P0_EndPosition_Num
  Bus Selector3 : BusSelector  OutputSignals=P0_dx_TrackRecord,P0_dy_TrackRecord,P0_Counter_TrackRecord,P0_StartPosition_Num,P0_EndPosition_Num
  If : If  IfExpression=u1 == 1
  Merge1 : Merge
  Merge2 : Merge
  Merge3 : Merge
  Relational Operator : RelationalOperator  Operator=<=  OutDataTypeStr=boolean  RndMeth=Simplest
  Relational Operator1 : RelationalOperator  Operator=>  OutDataTypeStr=boolean  RndMeth=Simplest
  Subsystem2 : Subsystem
  Subsystem3 : Subsystem
  Terminator : Terminator
  polyfit1 : MATLAB Function  Commented=on  TreatAsAtomicUnit=on
  dx : Outport
  dy : Outport  Port=2
  P0_Counter : Outport  Port=3
  wires:
  If/2 -> Subsystem3/Action
  If/1 -> Subsystem2/Action
  Bus Selector/1 -> Relational Operator/1  "<P0_StartPosition_Num>"
  Bus Selector/2 -> Relational Operator/2  "<P0_EndPosition_Num>"
  Relational Operator/1 -> If/1
  Relational Operator1/1 -> Terminator/1
  Bus Selector1/2 -> Relational Operator1/2  "<P0_EndPosition_Num>"
  Bus Selector1/1 -> Relational Operator1/1  "<P0_StartPosition_Num>"
  P0_TrackRecord/1 -> Bus Selector/1, Bus Selector1/1, [P0_TrackRecord]
  Subsystem2/1(dx) -> Merge3/1
  Merge3/1 -> dx/1
  Merge1/1 -> dy/1
  Merge2/1 -> P0_Counter/1
  Subsystem2/2(dy) -> Merge1/1
  Subsystem2/3(P0_Counter) -> Merge2/1
  Subsystem3/1(dx) -> Merge3/2
  Subsystem3/2(dy) -> Merge1/2
  Subsystem3/3(P0_Counter) -> Merge2/2
  [P0_TrackRecord] -> Bus Selector2/1
  Bus Selector2/1 -> Subsystem2/1(P0_dx_TrackRecord)  "<P0_dx_TrackRecord>"
  Bus Selector2/2 -> Subsystem2/2(P0_dy_TrackRecord)  "<P0_dy_TrackRecord>"
  Bus Selector2/3 -> Subsystem2/3(P0_Counter_TrackRecord)  "<P0_Counter_TrackRecord>"
  Bus Selector2/4 -> Subsystem2/4(P0_StartPosition_Num)  "<P0_StartPosition_Num>"
  Bus Selector2/5 -> Subsystem2/5(P0_EndPosition_Num)  "<P0_EndPosition_Num>"
  Bus Selector3/5 -> Subsystem3/5(P0_EndPosition_Num)  "<P0_EndPosition_Num>"
  Bus Selector3/4 -> Subsystem3/4(P0_StartPosition_Num)  "<P0_StartPosition_Num>"
  Bus Selector3/3 -> Subsystem3/3(P0_Counter_TrackRecord)  "<P0_Counter_TrackRecord>"
  Bus Selector3/2 -> Subsystem3/2(P0_dy_TrackRecord)  "<P0_dy_TrackRecord>"
  Bus Selector3/1 -> Subsystem3/1(P0_dx_TrackRecord)  "<P0_dx_TrackRecord>"
  [P0_TrackRecord] -> Bus Selector3/1

== system PubIfDecisionTOS_MDL/TOS_20201112/TOS_2012080320/TOS/P0_Trajectory_V1.0/TrackRecord ==
  note: 整数倍时，赋值
  note: 非整数倍时，赋值
  TOS_ACC_P0_Inf : Inport
  TrackRecord_CordinatConvert : Inport  Port=2
  Bus Creator : BusCreator  Inputs=9
  Bus Creator1 : BusCreator  Inputs=2
  Bus Selector3 : BusSelector  OutputSignals=TOS_ACC_P0_Inf.P0_Counter
  Compare To Constant : simulink/Logic and Bit Operations/Compare To Constant  relop=~=  const=uint32(0)  OutDataTypeStr=boolean
      settings: AttributesFormatString=P0_Invilad_Val = uint32(0)
  Compare To Constant1 : simulink/Logic and Bit Operations/Compare To Constant  relop=~=  const=uint32(0)  OutDataTypeStr=boolean
      settings: AttributesFormatString=P0_Invilad_Val = uint32(0)
  Compare To Constant2 : simulink/Logic and Bit Operations/Compare To Constant  relop===  const=uint32(0)  OutDataTypeStr=boolean
      settings: AttributesFormatString=P0_Invilad_Val = uint32(0)
  Constant1 : Constant  Value=P_TOS_P0_Trajectory_TrackRecord_Num  OutDataTypeStr=uint32
      settings: AttributesFormatString=P0_Trajectory_TrackRecord_Num = unit32(60)
  Constant3 : Constant  Value=P_TOS_P0_Trajectory_TrackRecord_Num  OutDataTypeStr=uint32
      settings: AttributesFormatString=P0_Trajectory_TrackRecord_Num = unit32(60)
  If : If  NumInputs=2  IfExpression=u1 == 1  ElseIfExpressions=u2 == 1
  Logical Operator1 : Logic  AllPortsSameDT=off  OutDataTypeStr=boolean
  Math Function : Math  Operator=mod  SaturateOnIntegerOverflow=on
  Merge{1..9} (9 alike) : Merge  Inputs=3
  Subsystem1 : Subsystem
  Subsystem2 : Subsystem
  Subsystem3 : Subsystem
  P0_TrackRecord : Outport
  wires:
  Subsystem1/5(P0_EndPosition_Num) -> Merge1/3
  Subsystem1/4(P0_StartPosition_Num) -> Merge5/3
  [P0_ModIndex_Sig] -> Subsystem3/1(P0_Index)
  Merge1/1 -> Bus Creator/5  "P0_EndPosition_Num"
  Merge5/1 -> Bus Creator/4  "P0_StartPosition_Num"
  Constant1/1 -> Subsystem2/1(P0_Index)
  [TrackRecord_CordinatConvert] -> Subsystem2/2(TrackRecord_Sig)
  If/1 -> Subsystem2/Action
  Logical Operator1/1 -> If/1
  Compare To Constant2/1 -> Logical Operator1/2
  Compare To Constant1/1 -> Logical Operator1/1
  Merge4/1 -> Bus Creator/2  "P0_dy_TrackRecord"
  Merge2/1 -> Bus Creator/3  "P0_Counter_TrackRecord"
  Subsystem1/2(P0_dy_TrackRecord) -> Merge4/3  "P0_dy_TrackRecord"
  Subsystem1/1(P0_dx_TrackRecord) -> Merge3/3  "P0_dx_TrackRecord"
  Subsystem1/3(P0_Counter_TrackRecord) -> Merge2/3  "P0_Counter_TrackRecord"
  Merge3/1 -> Bus Creator/1  "P0_dx_TrackRecord"
  Compare To Constant/1 -> If/2
  If/3 -> Subsystem1/Action
  [TrackRecord_CordinatConvert] -> Subsystem1/1(TrackRecord_Sig)
  Math Function/1 -> Compare To Constant2/1, [P0_ModIndex_Sig], Compare To Constant/1  "P0_Counter_Mod"
  If/2 -> Subsystem3/Action
  [TrackRecord_CordinatConvert] -> Subsystem3/2(TrackRecord_Sig)
  Bus Selector3/1 -> Compare To Constant1/1, Math Function/1  "<P0_Counter>"
  Bus Creator1/1 -> Bus Selector3/1, [TrackRecord_CordinatConvert]
  TrackRecord_CordinatConvert/1 -> Bus Creator1/2
  Constant3/1 -> Math Function/2
  TOS_ACC_P0_Inf/1 -> Bus Creator1/1
  Bus Creator/1 -> P0_TrackRecord/1
  Subsystem1/6(P0_ID_TrackRecord) -> Merge6/3
  Merge6/1 -> Bus Creator/6  "P0_ID_TrackRecord"
  Subsystem1/7(P0_StartPosition_Dis) -> Merge7/2
  Subsystem1/8(P0_EndPosition_dx) -> Merge8/2
  Merge7/1 -> Bus Creator/7  "P0_StartPosition_Dis"
  Merge8/1 -> Bus Creator/8  "P0_EndPosition_dx"
  Subsystem1/9(P0_EndPosition_dy) -> Merge9/2
  Merge9/1 -> Bus Creator/9  "P0_EndPosition_dy"
  Subsystem2/1(P0_dx_TrackRecord) -> Merge3/1
  Subsystem2/2(P0_dy_TrackRecord) -> Merge4/1
  Subsystem2/3(P0_Counter_TrackRecord) -> Merge2/1
  Subsystem2/4(P0_StartPosition_Num) -> Merge5/1
  Subsystem2/5(P0_EndPosition_Num) -> Merge1/1
  Subsystem2/6(P0_ID_TrackRecord) -> Merge6/1
  Subsystem2/7(P0_StartPosition_Dis) -> Merge7/1
  Subsystem2/8(P0_EndPosition_dx) -> Merge8/1
  Subsystem2/9(P0_EndPosition_dy) -> Merge9/1
  Subsystem3/1(P0_dx_TrackRecord) -> Merge3/2
  Subsystem3/2(P0_dy_TrackRecord) -> Merge4/2
  Subsystem3/3(P0_Counter_TrackRecord) -> Merge2/2
  Subsystem3/4(P0_StartPosition_Num) -> Merge5/2
  Subsystem3/5(P0_EndPosition_Num) -> Merge1/2
  Subsystem3/6(P0_ID_TrackRecord) -> Merge6/2
  Subsystem3/7(P0_StartPosition_Dis) -> Merge7/3
  Subsystem3/8(P0_EndPosition_dx) -> Merge8/3
  Subsystem3/9(P0_EndPosition_dy) -> Merge9/3

== system PubIfDecisionTOS_MDL/TOS_20201112/TOS_2012080320/TOS/P0_Trajectory_V1.0/TrgValidConfirm ==
  TOS_ACC_P0 : Inport
  Signal Copy : SignalConversion  OverrideOpt=off
  TrgValidConfirm : Subsystem
  Unit Delay1 : UnitDelay  InitialCondition=uint8(0)  SampleTime=-1  HasFrameUpgradeWarning=on
  Unit Delay3 : UnitDelay  InitialCondition=uint8(0)  SampleTime=-1  HasFrameUpgradeWarning=on
  Unit Delay4 : UnitDelay  InitialCondition=uint8(0)  SampleTime=-1  HasFrameUpgradeWarning=on
  P0_ID : Outport
  P0_Counter : Outport  Port=2
  P0_dx : Outport  Port=3
  P0_dy : Outport  Port=4
  wires:
  Unit Delay1/1 -> TrgValidConfirm/3(P0_dx_K1)
  TrgValidConfirm/1(P0_ID) -> Unit Delay3/1, P0_ID/1  "P0_ID"
  Unit Delay3/1 -> TrgValidConfirm/1(P0_ID_K1)
  TrgValidConfirm/4(P0_dy) -> P0_dy/1  "P0_dy"
  Unit Delay4/1 -> TrgValidConfirm/2(P0_Counter_K1)
  TrgValidConfirm/3(P0_dx) -> P0_dx/1, Unit Delay1/1  "P0_dx"
  TrgValidConfirm/2(P0_Counter) -> Unit Delay4/1, Signal Copy/1  "TOS_P0_TARGET_TrgValidConfirm_P0_Counter_ObserVale"
  TOS_ACC_P0/1 -> TrgValidConfirm/4(TOS_ACC_P0)
  Signal Copy/1 -> P0_Counter/1  "P0_Counter"

== system PubIfDecisionTOS_MDL/TOS_20201112/TOS_2012080320/PIL_1029/BoundaryCalculat/Lane_BoundaryCalculat/Lane_Boundary ==
  TOS_OFMObjValid_Flag : Inport  Partition=on  PartitionDimension=1  PartitionWidth=1  PartitionOffset=0
  Object_Type : Inport  Port=2  Partition=on  PartitionDimension=1  PartitionWidth=1  PartitionOffset=0
  Object_DX : Inport  Port=3  Partition=on  PartitionDimension=1  PartitionWidth=1  PartitionOffset=0
  object_MovingState : Inport  Port=4  Partition=on  PartitionDimension=1  PartitionWidth=1  PartitionOffset=0
  PP_CurrentLaneWidth : Inport  Port=5
  PP_LeftLaneWidth : Inport  Port=6
  PP_RightLaneWidth : Inport  Port=7
  C_LaneLineCourseErrorFront : Inport  Port=8
  C_LaneLineCourseErrorRear : Inport  Port=9
  Boundary : Subsystem
  BoundaryDefault : Subsystem  TreatAsAtomicUnit=on
  Compare To Constant : simulink/Logic and Bit Operations/Compare To Constant  relop===  const=C_TOS_OFMObjIDInvilad_Val  OutDataTypeStr=boolean
      settings: AttributesFormatString=C_TOS_OFMObjIDInvilad_Val = 0
  For Each : ForEach  DisableCoverage=on
  If : If  IfExpression=u1 ~= 0
  Merge{,1..11} (12 alike) : Merge
  SameLane_CoreArea_Boundary : Outport  ConcatenationDimension=1
  SameLane_EdgeLeft_Boundary : Outport  Port=2  ConcatenationDimension=1
  SameLane_EdgeRight_Boundary : Outport  Port=3  ConcatenationDimension=1
  LeftLane_CoreArea_Boundary : Outport  Port=4  ConcatenationDimension=1
  LeftLane_EdgeLeft_Boundary : Outport  Port=5  ConcatenationDimension=1
  LeftLane_EdgeRight_Boundary : Outport  Port=6  ConcatenationDimension=1
  RightLane_CoreArea_Boundary : Outport  Port=7  ConcatenationDimension=1
  RightLane_EdgeLeft_Boundary : Outport  Port=8  ConcatenationDimension=1
  RightLane_EdgeRight_Boundary : Outport  Port=9  ConcatenationDimension=1
  SameLane_BasicLaneWidth_ObserVale : Outport  Port=10  ConcatenationDimension=1
  LeftLane_BasicLaneWidth_ObserVale : Outport  Port=11  ConcatenationDimension=1
  RightLane_BasicLaneWidth_ObserVale : Outport  Port=12  ConcatenationDimension=1
  wires:
  Merge11/1 -> RightLane_BasicLaneWidth_ObserVale/1
  Merge10/1 -> LeftLane_BasicLaneWidth_ObserVale/1
  Merge9/1 -> SameLane_BasicLaneWidth_ObserVale/1
  BoundaryDefault/12(RightLane_BasicLaneWidth_ObserVale) -> Merge11/1
  BoundaryDefault/11(LeftLane_BasicLaneWidth_ObserVale) -> Merge10/1
  BoundaryDefault/10(SameLane_BasicLaneWidth_ObserVale) -> Merge9/1
  Boundary/12(RightLane_BasicLaneWidth_ObserVale) -> Merge11/2
  Boundary/11(LeftLane_BasicLaneWidth_ObserVale) -> Merge10/2
  Boundary/10(SameLane_BasicLaneWidth_ObserVale) -> Merge9/2
  BoundaryDefault/9(RightLane_EdgeRight_Boundary) -> Merge8/1
  BoundaryDefault/8(RightLane_EdgeLeft_Boundary) -> Merge7/1
  BoundaryDefault/7(RightLane_CoreArea_Boundary) -> Merge6/1
  BoundaryDefault/6(LeftLane_EdgeRight_Boundary) -> Merge5/1
  BoundaryDefault/5(LeftLane_EdgeLeft_Boundary) -> Merge4/1
  Boundary/5(LeftLane_EdgeLeft_Boundary) -> Merge4/2
  Boundary/6(LeftLane_EdgeRight_Boundary) -> Merge5/2
  Boundary/7(RightLane_CoreArea_Boundary) -> Merge6/2
  Boundary/8(RightLane_EdgeLeft_Boundary) -> Merge7/2
  Boundary/9(RightLane_EdgeRight_Boundary) -> Merge8/2
  Boundary/4(LeftLane_CoreArea_Boundary) -> Merge3/2
  BoundaryDefault/4(LeftLane_CoreArea_Boundary) -> Merge3/1
  Merge8/1 -> RightLane_EdgeRight_Boundary/1
  Merge7/1 -> RightLane_EdgeLeft_Boundary/1
  Merge6/1 -> RightLane_CoreArea_Boundary/1
  Merge3/1 -> LeftLane_CoreArea_Boundary/1
  Merge4/1 -> LeftLane_EdgeLeft_Boundary/1
  Merge5/1 -> LeftLane_EdgeRight_Boundary/1
  PP_RightLaneWidth/1 -> Boundary/6(PP_RightLaneWidth)  "PP_RightLaneWidth"
  PP_LeftLaneWidth/1 -> Boundary/5(PP_LeftLaneWidth)  "PP_LeftLaneWidth"
  Merge2/1 -> SameLane_EdgeRight_Boundary/1
  Merge1/1 -> SameLane_EdgeLeft_Boundary/1
  Merge/1 -> SameLane_CoreArea_Boundary/1
  BoundaryDefault/3(SameLane_EdgeRight_Boundary) -> Merge2/1
  BoundaryDefault/2(SameLane_EdgeLeft_Boundary) -> Merge1/1
  BoundaryDefault/1(SameLane_CoreArea_Boundary) -> Merge/1
  If/2 -> Boundary/Action
  If/1 -> BoundaryDefault/Action
  TOS_OFMObjValid_Flag/1 -> Compare To Constant/1
  Compare To Constant/1 -> If/1
  Boundary/3(SameLane_EdgeRight_Boundary) -> Merge2/2
  Boundary/2(SameLane_EdgeLeft_Boundary) -> Merge1/2
  Boundary/1(SameLane_CoreArea_Boundary) -> Merge/2
  C_LaneLineCourseErrorRear/1 -> Boundary/8(C_LaneLineCourseErrorRear)  "C_LaneLineCourseErrorRear"
  C_LaneLineCourseErrorFront/1 -> Boundary/7(C_LaneLineCourseErrorFront)  "C_LaneLineCourseErrorFront"
  PP_CurrentLaneWidth/1 -> Boundary/4(PP_CurrentLaneWidth)  "PP_CurrentLaneWidth"
  object_MovingState/1 -> Boundary/3(object_MovingState)  "object_MovingState"
  Object_DX/1 -> Boundary/2(Object_DX)  "Object_DX"
  Object_Type/1 -> Boundary/1(Object_Type)  "Object_Type"

== system PubIfDecisionTOS_MDL/TOS_20201112/TOS_2012080320/PIL_1029/BoundaryCalculat/ObjectToCenterLine_dyc/LeftLane ==
  Left_CenterLine : Inport
  OFM_SignalVerification : Inport  Port=2
  Bus Selector : BusSelector  OutputSignals=TOS_OFMObjValid_Flag,Object_ID,Object_Age
  Bus Selector3 : BusSelector  OutputSignals=CenterLine01.PC0,CenterLine01.PC1,CenterLine01.PC2,CenterLine01.PC3,CenterLine01.dDisStart,CenterLine01.dDisEnd,CenterLine02.PC0,CenterLine02.PC1,CenterLine02.PC2,CenterLine02.PC3,CenterLine02.dDisStart,CenterLine02.dDisEnd,CenterLine03.PC0,CenterLine03.PC1,CenterLine03.PC2,CenterLine03.PC3,CenterLine03.dDisStart,CenterLine03.dDisEnd,CenterLine04.PC0,CenterLine04.PC1,CenterLine04.PC2,CenterLine04.PC3,CenterLine04.dDisStart,CenterLine04.dDisEnd,CenterLine05.PC0,CenterLine05.PC1,CenterLine05.PC2,CenterLine05.PC3,CenterLine05.dDisStart,CenterLine05.dDisEnd,CenterLine06.PC0,CenterLine06.PC1,CenterLine06.PC2,CenterLine06.PC3,CenterLine06.dDisStart,CenterLine06.dDisEnd
  Bus Selector4 : BusSelector  OutputSignals=TOS_OFMObjValid_Flag,Object_DY,Object_DX
  LeftCenterLine_dyc : Subsystem
  PIL_ObjectToCenterLine_dy_Filt : Subsystem
  PIL_LeftCenterLine_dyc : Outport
  PIL_LeftCenterLine_dyc_Filt : Outport  Port=2
  wires:
  LeftCenterLine_dyc/1(LeftCenterLine_dyc) -> PIL_ObjectToCenterLine_dy_Filt/4(ObjectToCenterLine_dy), PIL_LeftCenterLine_dyc/1
  Bus Selector3/2 -> LeftCenterLine_dyc/5(line01_C1)  "<PC1>"
  Bus Selector3/3 -> LeftCenterLine_dyc/6(line01_C2)  "<PC2>"
  Bus Selector3/4 -> LeftCenterLine_dyc/7(line01_C3)  "<PC3>"
  Bus Selector3/7 -> LeftCenterLine_dyc/10(line02_C0)  "<PC0>"
  Bus Selector3/5 -> LeftCenterLine_dyc/8(line01_dDisStart)  "<dDisStart>"
  Bus Selector4/3 -> LeftCenterLine_dyc/3(Object_DX)  "<Object_DX>"
  Bus Selector3/12 -> LeftCenterLine_dyc/15(line02_dDisEnd)  "<dDisEnd>"
  Bus Selector3/18 -> LeftCenterLine_dyc/21(line03_dDisEnd)  "<dDisEnd>"
  Bus Selector3/36 -> LeftCenterLine_dyc/39(line06_dDisEnd)  "<dDisEnd>"
  Bus Selector3/19 -> LeftCenterLine_dyc/22(line04_C0)  "<PC0>"
  Bus Selector3/13 -> LeftCenterLine_dyc/16(line03_C0)  "<PC0>"
  Bus Selector4/2 -> LeftCenterLine_dyc/2(Object_DY)  "<Object_DY>"
  Bus Selector3/23 -> LeftCenterLine_dyc/26(line04_dDisStart)  "<dDisStart>"
  Bus Selector3/15 -> LeftCenterLine_dyc/18(line03_C2)  "<PC2>"
  Bus Selector3/24 -> LeftCenterLine_dyc/27(line04_dDisEnd)  "<dDisEnd>"
  Bus Selector3/29 -> LeftCenterLine_dyc/32(line05_dDisStart)  "<dDisStart>"
  Bus Selector3/11 -> LeftCenterLine_dyc/14(line02_dDisStart)  "<dDisStart>"
  Bus Selector3/26 -> LeftCenterLine_dyc/29(line05_C1)  "<PC1>"
  Bus Selector3/17 -> LeftCenterLine_dyc/20(line03_dDisStart)  "<dDisStart>"
  Bus Selector3/21 -> LeftCenterLine_dyc/24(line04_C2)  "<PC2>"
  Bus Selector3/30 -> LeftCenterLine_dyc/33(line05_dDisEnd)  "<dDisEnd>"
  Bus Selector3/20 -> LeftCenterLine_dyc/23(line04_C1)  "<PC1>"
  Bus Selector3/27 -> LeftCenterLine_dyc/30(line05_C2)  "<PC2>"
  Bus Selector3/32 -> LeftCenterLine_dyc/35(line06_C1)  "<PC1>"
  Bus Selector3/28 -> LeftCenterLine_dyc/31(line05_C3)  "<PC3>"
  Bus Selector3/1 -> LeftCenterLine_dyc/4(line01_C0)  "<PC0>"
  Bus Selector3/14 -> LeftCenterLine_dyc/17(line03_C1)  "<PC1>"
  Bus Selector3/10 -> LeftCenterLine_dyc/13(line02_C3)  "<PC3>"
  Bus Selector3/33 -> LeftCenterLine_dyc/36(line06_C2)  "<PC2>"
  Bus Selector4/1 -> LeftCenterLine_dyc/1(TOS_OFMObjValid_Flag)  "<TOS_OFMObjValid_Flag>"
  Bus Selector3/8 -> LeftCenterLine_dyc/11(line02_C1)  "<PC1>"
  Bus Selector3/16 -> LeftCenterLine_dyc/19(line03_C3)  "<PC3>"
  Bus Selector3/31 -> LeftCenterLine_dyc/34(line06_C0)  "<PC0>"
  Bus Selector3/22 -> LeftCenterLine_dyc/25(line04_C3)  "<PC3>"
  Bus Selector3/6 -> LeftCenterLine_dyc/9(line01_dDisEnd)  "<dDisEnd>"
  Bus Selector3/9 -> LeftCenterLine_dyc/12(line02_C2)  "<PC2>"
  Bus Selector3/25 -> LeftCenterLine_dyc/28(line05_C0)  "<PC0>"
  Bus Selector3/35 -> LeftCenterLine_dyc/38(line06_dDisStart)  "<dDisStart>"
  Bus Selector3/34 -> LeftCenterLine_dyc/37(line06_C3)  "<PC3>"
  Left_CenterLine/1 -> Bus Selector3/1
  OFM_SignalVerification/1 -> [OFM_SignalVerification], Bus Selector4/1
  [OFM_SignalVerification] -> Bus Selector/1
  Bus Selector/1 -> PIL_ObjectToCenterLine_dy_Filt/1(TOS_OFMObjValid_Flag)  "<TOS_OFMObjValid_Flag>"
  Bus Selector/2 -> PIL_ObjectToCenterLine_dy_Filt/2(Object_ID)  "<Object_ID>"
  Bus Selector/3 -> PIL_ObjectToCenterLine_dy_Filt/3(Object_Age)  "<Object_Age>"
  PIL_ObjectToCenterLine_dy_Filt/1(PIL_ObjectToCenterLine_dy_Filt) -> PIL_LeftCenterLine_dyc_Filt/1
